simulink model "sedemo_DVS_model"  (Simulink 7.5)
settings: Solver=VariableStepDiscrete  StartTime=0.0  StopTime=inf  MaxStep=inf  RelTol=1e-3
undefined symbols (not defined in the file or in its folder): des_subsystemblock, des_subsysteminport, des_subsystemoutport, des_subsystemsupportblock, sedemo_DVS_gain_fcn, sedemo_DVS_init_fcn
libraries: simeventstranslate1 x3, simeventsgenerators1 x3, simulink x2, simeventssignalmanage1 x2, simeventstiming1 x2, simeventssink1 x1, simeventsqueue1 x1, simeventsserver1 x1, simeventsgates1 x1
settings Model: Creator=The MathWorks Inc.  ExtModeAutoUpdateStatusClock=off
settings DataIOCC: SaveOutput=off  SignalLogging=off  SaveTime=off
settings OptimizationCC: InitFltsAndDblsToZero=on
settings DebuggingCC: AlgebraicLoopMsg=error  SaveWithParameterizedLinksMsg=none  SignalResolutionControl=TryResolveAllWithWarning  SolverPrmCheckMsg=none  MultiTaskDSMMsg=warning  MultiTaskCondExecSysMsg=none  StrictBusMsg=Warning
settings RTWCC: IncludeERTFirstTime=on
settings GRTTargetCC: TargetFcnLib=ansi_tfl_tmw.mat
settings SimEventsCC: propIdentEventSeed=12345678  propDiagAttribOutput=1  propDiagFcnCallOutput=1  propDiagStatOutput=0

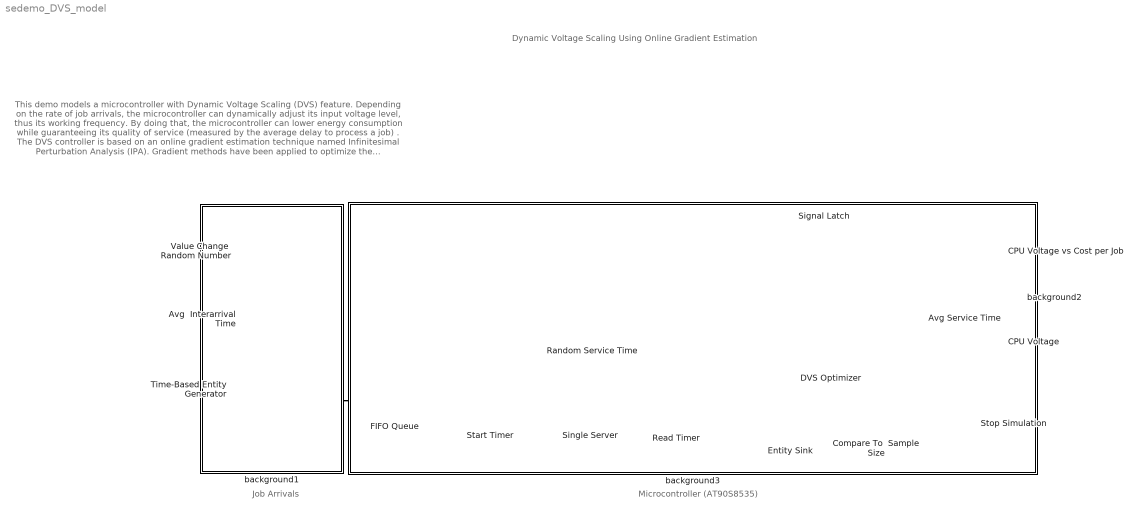
== system sedemo_DVS_model ==
  note: Job Arrivals
  note: Microcontroller (AT90S8535)
  note: Dynamic Voltage Scaling Using Online Gradient Estimation
  note: This demo models a microcontroller with Dynamic Voltage Scaling (DVS) feature. Depending on the rate of job arrivals, the microcontroller can dynamically
      | adjust its input voltage level, thus its working frequency. By doing that, the microcontroller can lower energy consumption while guaranteeing its quality
      | of service (measured by the average delay to process a job) .
      |
      | The DVS controller is based on an online gradient estimation technique named Infinitesimal Perturbation Analysis (IPA). Gradient methods have been applied
      | to optimize the performance of the microcontroller.
      |
      | During the simulation, observe how the DVS controller finds the optimal input voltage. Try changing the Avg Interarrival Time to values between 0.15 and
      | 3.0 when running the model.
  Avg  Interarrival Time : Subsystem  LoadFcn=slideg Load  InitFcn=|  StartFcn=slideg StartFcn  StopFcn=slideg StopFcn  mask(Slider Gain){low=0.15, gain=0.26, high=3}
      | global int_arr;                        
      | int_arr=str2num(get_param(gcb,'gain'));
      settings: CopyFcn=slideg Copy  DeleteFcn=slideg DeleteBlock  NameChangeFcn=slideg NameChange  OpenFcn=slideg Open  CloseFcn=slideg Close  ParentCloseFcn=slideg ParentClose
      mask Display: disp(gain)
  Avg Service Time : Display
  CPU Voltage : Display
  CPU Voltage vs Cost per Job : MATLABFcn  LoadFcn=|  StartFcn=sedemo_DVS_init_fcn;  MATLABFcn=sedemo_DVS_plot_fcn  OutputDimensions=0
      | global FigureHdl;
      | FigureHdl=1;
      settings: ModelCloseFcn=|
      | global FigureHdl;
      | figure(FigureHdl);
      | close(FigureHdl);
      | clear tout;
      | clear global FigureHdl;
      | clear int_arr;
  Compare To  Sample Size : simulink/Logic and Bit Operations/Compare To Constant  SystemSampleTime=-1  relop=>  const=5000  LogicOutDataTypeMode=boolean  ZeroCross=off
  DVS Optimizer : Subsystem
  Entity Sink : simeventssink1/Entity Sink  Priority=1  SystemSampleTime=-1  AvailableForArrivals=on  StatNumberArrived=On
  FIFO Queue : simeventsqueue1/FIFO Queue  Priority=1  SystemSampleTime=-1  Capacity=1e10  EnableTOPort=off  StatNumberDeparted=Off  StatNumberInBlock=On  StatPendingEntity=Off  StatAverageWait=Off  StatAverageQueueLength=Off  StatNumberTimedout=Off
  Random Service Time : Subsystem
  Read Timer : simeventstiming1/Read Timer  Priority=0  SystemSampleTime=-1  TimerTag=T1  TimerModeOption=Error  TimerStop=off  StatNumberDeparted=On  StatTimerNumberDeparted=Off  StatTimeElapsed=On  StatAverageTimeElapsed=Off
  Signal Latch : simeventssignalmanage1/Signal Latch  Priority=1  SystemSampleTime=-1  InitialMemoryValue=0.125  WriteMemoryUpon=Change in signal from port wvc  MemoryWriteEdgeOption=Either  SpecifyWriteEventPriority=off  PriorityMemoryWrite=7100  ReadMemoryUpon=Write to memory event  MemoryReadEdgeOption=Falling  SpecifyReadEventPriority=on  PriorityMemoryRead=7000  ReportMemoryState=off  ReportMemoryUponWrite=off  ReportMemoryUponRead=on
  Single Server : simeventsserver1/Single Server  Priority=1  SystemSampleTime=-1  ServiceTimeFrom=Signal port t  ServiceTime=1  AttributeName=ServiceTime  PriorityServiceCompletion=500  PermitPreemption=off  SortingAttributeName=PriorityAttributeName  SortingDirection=Ascending  WriteToAttribute=off  ResidualAttributeName=ResidualServiceTime  CreateAttribute=on  EnableTOPort=off  StatNumberDeparted=Off  StatNumberInBlock=Off  StatNumberPreempted=Off  StatPendingEntity=Off  StatAverageWait=Off  StatUtilization=Off  StatNumberTimedout=Off
  Start Timer : simeventstiming1/Start Timer  Priority=0  SystemSampleTime=-1  TimerTag=T1  TimerStartedOption=Warn and continue  StatNumberDeparted=On
  Stop Simulation : Stop
  Time-Based Entity Generator : simeventsgenerators1/Entity Generators/Time-Based Entity Generator  Priority=1  DialogController=des_ddg_create  DialogControllerArgs=DataTag18  SystemSampleTime=-1  GenerateEntitiesUpon=Intergeneration time from port t  Distribution=Constant  Minimum=0  Maximum=1  Mean=1  InitialSeed=12345  Period=1  PriorityEntityGeneration=300  GenerateEntityAtSimulationStart=off  ResponseWhenBlocked=Pause generation  ResponseWhenUnblocked=Immediate restart  EntityType=Standard  StatNumberDeparted=On  StatPendingEntity=Off  StatAverageIntergenerationTime=Off
  Value Change  Random Number : Subsystem
  background1 : Subsystem
      mask Display: disp('')
  background2 : Subsystem
      mask Display: disp('')
  background3 : Subsystem
      mask Display: disp('')
  wires:
  Read Timer/1 -> DVS Optimizer/3(#d)
  DVS Optimizer/2(voltage) -> CPU Voltage/1
  Signal Latch/1 -> DVS Optimizer/2(theta0), Random Service Time/1(in)
  DVS Optimizer/1(theta1) -> Avg Service Time/1, Signal Latch/2, Signal Latch/1, CPU Voltage vs Cost per Job/1
  FIFO Queue/1 -> DVS Optimizer/1(QState)
  Value Change  Random Number/1(out) -> Avg  Interarrival Time/1(In1)
  Random Service Time/1(out) -> Single Server/1
  Read Timer/2 -> DVS Optimizer/4(et)
  Start Timer/1 -> Random Service Time/2(vc)
  Entity Sink/1 -> Compare To  Sample Size/1
  Avg  Interarrival Time/1(Out1) -> Time-Based Entity Generator/1
  Time-Based Entity Generator/1 -> Value Change  Random Number/1(vc)
  Compare To  Sample Size/1 -> Stop Simulation/1
  connections:
  FIFO Queue/RConn1 -- Start Timer/LConn1
  Start Timer/RConn1 -- Single Server/LConn1
  Single Server/RConn1 -- Read Timer/LConn1
  Read Timer/RConn1 -- Entity Sink/LConn1
  Time-Based Entity Generator/RConn1 -- FIFO Queue/LConn1

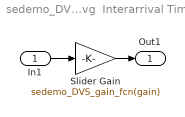
== system sedemo_DVS_model/Avg  Interarrival Time ==
  In1 : Inport  OutDataType=sfix(16)  OutScaling=2^0
  Slider Gain : Gain  Gain=sedemo_DVS_gain_fcn(gain)  ParameterDataType=sfix(16)  ParameterScaling=2^0  OutDataType=sfix(16)  OutScaling=2^0  SaturateOnIntegerOverflow=on  OutDataTypeStr=Inherit: Same as input  ParamDataTypeStr=Inherit: Same as input
  Out1 : Outport  OutDataType=sfix(16)  OutScaling=2^0
  wires:
  Slider Gain/1 -> Out1/1
  In1/1 -> Slider Gain/1

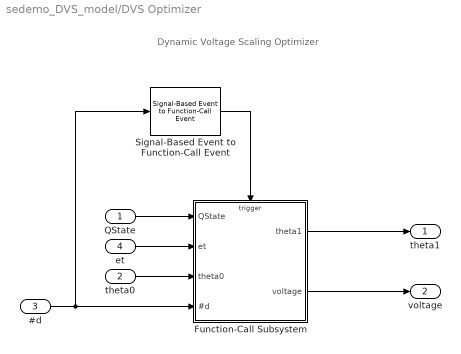
== system sedemo_DVS_model/DVS Optimizer ==
  note: Dynamic Voltage Scaling Optimizer
  QState : Inport  OutDataType=sfix(16)  OutScaling=2^0
  theta0 : Inport  Port=2  OutDataType=sfix(16)  OutScaling=2^0
  #d : Inport  Port=3  OutDataType=sfix(16)  OutScaling=2^0
  et : Inport  Port=4  OutDataType=sfix(16)  OutScaling=2^0
  Function-Call Subsystem : Subsystem  TreatAsAtomicUnit=on
      settings: PropExecContextOutsideSubsystem=on
  Signal-Based Event to Function-Call Event : simeventstranslate1/Signal-Based Event to Function-Call Event  Priority=1  SystemSampleTime=-1  GenerateFunctionCallUpon=Change in signal from port vc  SignalEdgeOption=Rising  EnableE1Port=off  EnableF2Port=off  EnableE2Port=off  SpecifyEventPriority=off  PriorityFunctionCall=200  FunctionCallDelayFrom=Dialog  DelayFunctionCall=0  StatNumberF1Calls=Off  StatNumberF2Calls=Off
  theta1 : Outport  OutDataType=sfix(16)  OutScaling=2^0
  voltage : Outport  Port=2  OutDataType=sfix(16)  OutScaling=2^0
  wires:
  Signal-Based Event to Function-Call Event/1 -> Function-Call Subsystem/Trigger
  #d/1 -> Signal-Based Event to Function-Call Event/1, Function-Call Subsystem/4(#d)
  QState/1 -> Function-Call Subsystem/1(QState)
  et/1 -> Function-Call Subsystem/2(et)
  theta0/1 -> Function-Call Subsystem/3(theta0)
  Function-Call Subsystem/1(theta1) -> theta1/1
  Function-Call Subsystem/2(voltage) -> voltage/1

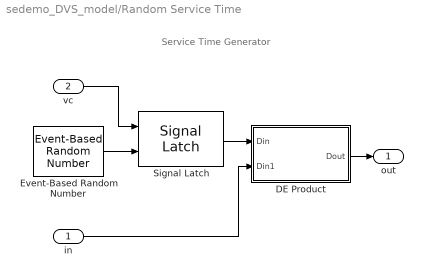
== system sedemo_DVS_model/Random Service Time ==
  note: Service Time Generator
  in : Inport  OutDataType=sfix(16)  OutScaling=2^0
  vc : Inport  Port=2  OutDataType=sfix(16)  OutScaling=2^0
  DE Product : Subsystem  LoadFcn=des_subsystemblock(gcb, 'load');  InitFcn=des_subsystemblock(gcb, 'init');  StartFcn=des_subsystemblock(gcb, 'start');  StopFcn=des_subsystemblock(gcb, 'stop');
      settings: CopyFcn=des_subsystemblock(gcb, 'copy');  DeleteFcn=des_subsystemblock(gcb, 'delete');  UndoDeleteFcn=des_subsystemblock(gcb, 'undodelete');  ModelCloseFcn=des_subsystemblock(gcb, 'modelclose');  PreSaveFcn=des_subsystemblock(gcb, 'presave');  NameChangeFcn=des_subsystemblock(gcb, 'namechange');  OpenFcn=des_subsystemblock(gcb, 'open');  ParentCloseFcn=des_subsystemblock(gcb, 'parentclose');  ErrorFcn=des_subsystemerror
      mask Type: Discrete Event Subsystem
      mask Help: helpview(simeventsbhelp);
  Event-Based Random Number : simeventsgenerators1/Signal Generators/Event-Based Random Number  SystemSampleTime=-1  distribution=Exponential  meanExp=1  minUnif=0  maxUnif=1  pOneBern=0.25  pSuccessBino=0.5  numTrialBino=1  meanNorm=0  stdNorm=1  minTri=1  maxTri=3  modeTri=2  thresholdLogn=0  scaleLogn=1  shapeLogn=1  pSuccessGeo=0.5  meanPoiss=1  thresholdLogl=0  scaleLogl=1  thresholdGam=0  scaleGam=1  shapeGam=1  minBeta=0  maxBeta=1  shape1Beta=1  shape2Beta=1  minUnid=0  maxUnid=1  numValueUnid=2  thresholdWbl=0  scaleWbl=1  shapeWbl=1  valueVecCont=[0 1]  cdfVecCont=[0 1]  valueVecDisc=[0 1]  probVecDisc=[0.5 0.5]  seed=35467  IsProcessed=on  isConnected=1
  Signal Latch : simeventssignalmanage1/Signal Latch  Priority=1  SystemSampleTime=-1  InitialMemoryValue=.22  WriteMemoryUpon=Change in signal from port wvc  MemoryWriteEdgeOption=Rising  SpecifyWriteEventPriority=on  PriorityMemoryWrite=7100  ReadMemoryUpon=Write to memory event  MemoryReadEdgeOption=Falling  SpecifyReadEventPriority=on  PriorityMemoryRead=7000  ReportMemoryState=off  ReportMemoryUponWrite=off  ReportMemoryUponRead=on
  out : Outport  OutDataType=sfix(16)  OutScaling=2^0
  wires:
  DE Product/1(Dout) -> out/1
  Event-Based Random Number/1 -> Signal Latch/2
  vc/1 -> Signal Latch/1
  Signal Latch/1 -> DE Product/1(Din)
  in/1 -> DE Product/2(Din1)

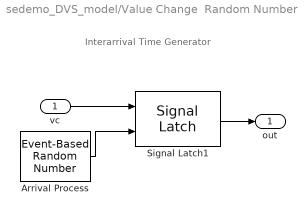
== system sedemo_DVS_model/Value Change  Random Number ==
  note: Interarrival Time Generator
  vc : Inport  OutDataType=sfix(16)  OutScaling=2^0
  Arrival Process : simeventsgenerators1/Signal Generators/Event-Based Random Number  SystemSampleTime=-1  distribution=Exponential  meanExp=1  minUnif=0  maxUnif=1  pOneBern=0.25  pSuccessBino=0.5  numTrialBino=1  meanNorm=0  stdNorm=1  minTri=1  maxTri=3  modeTri=2  thresholdLogn=0  scaleLogn=1  shapeLogn=1  pSuccessGeo=0.5  meanPoiss=1  thresholdLogl=0  scaleLogl=1  thresholdGam=0  scaleGam=1  shapeGam=1  minBeta=0  maxBeta=1  shape1Beta=1  shape2Beta=1  minUnid=0  maxUnid=1  numValueUnid=2  thresholdWbl=0  scaleWbl=1  shapeWbl=1  valueVecCont=[0 1]  cdfVecCont=[0 1]  valueVecDisc=[0 1]  probVecDisc=[0.5 0.5]  seed=98765  IsProcessed=on  isConnected=1
  Signal Latch1 : simeventsgates1/Signal Latch  Priority=1  SystemSampleTime=-1  InitialMemoryValue=0.45  WriteMemoryUpon=Change in signal from port wvc  MemoryWriteEdgeOption=Rising  SpecifyWriteEventPriority=on  PriorityMemoryWrite=7100  ReadMemoryUpon=Write to memory event  MemoryReadEdgeOption=Falling  SpecifyReadEventPriority=on  PriorityMemoryRead=7000  ReportMemoryState=off  ReportMemoryUponWrite=off  ReportMemoryUponRead=on
  out : Outport  OutDataType=sfix(16)  OutScaling=2^0
  wires:
  Arrival Process/1 -> Signal Latch1/2
  vc/1 -> Signal Latch1/1
  Signal Latch1/1 -> out/1

== system sedemo_DVS_model/background1 ==

== system sedemo_DVS_model/background2 ==

== system sedemo_DVS_model/background3 ==

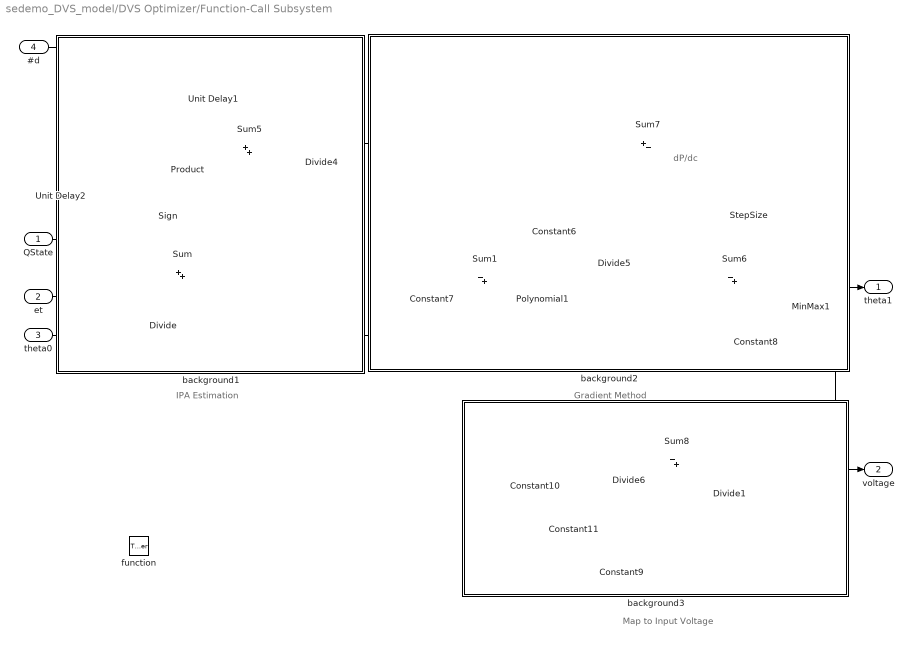
== system sedemo_DVS_model/DVS Optimizer/Function-Call Subsystem ==
  note: Map to Input Voltage
  note: dP/dc
  note: Gradient Method
  note: IPA Estimation
  QState : Inport  OutDataType=sfix(16)  OutScaling=2^0
  et : Inport  Port=2  OutDataType=sfix(16)  OutScaling=2^0
  theta0 : Inport  Port=3  OutDataType=sfix(16)  OutScaling=2^0
  #d : Inport  Port=4  OutDataType=sfix(16)  OutScaling=2^0
  function : TriggerPort  TriggerType=function-call
  Constant10 : Constant  Value=1/12  OutDataType=sfix(16)  OutScaling=2^0
  Constant11 : Constant  OutDataType=sfix(16)  OutScaling=2^0
  Constant6 : Constant  Value=1/36  OutDataType=sfix(16)  OutScaling=2^0
  Constant7 : Constant  Value=1/12  OutDataType=sfix(16)  OutScaling=2^0
  Constant8 : Constant  Value=0.12  OutDataType=sfix(16)  OutScaling=2^0
  Constant9 : Constant  Value=2  OutDataType=sfix(16)  OutScaling=2^0
  Divide : Product  Inputs=*/  OutDataType=sfix(16)  OutScaling=2^-10
  Divide1 : Product  Inputs=/*  OutDataType=sfix(16)  OutScaling=2^-10
  Divide4 : Product  Inputs=/*  OutDataType=sfix(16)  OutScaling=2^-10
  Divide5 : Product  Inputs=**/  OutDataType=sfix(16)  OutScaling=2^-10
  Divide6 : Product  Inputs=/*  OutDataType=sfix(16)  OutScaling=2^-10
  MinMax1 : MinMax  Function=max  Inputs=2  OutDataType=sfix(16)  OutScaling=2^0
  Polynomial1 : simulink/Math Operations/Polynomial  coefs=[1,0,0,0]
  Product : Product  OutDataType=sfix(16)  OutScaling=2^0  RndMeth=Zero
  Sign : Signum
  StepSize : Gain  Gain=1e-5  ParameterDataType=sfix(16)  ParameterScaling=2^0  OutDataType=sfix(16)  OutScaling=2^0
  Sum : Sum  Inputs=|++  OutDataType=sfix(16)  OutScaling=2^0
  Sum1 : Sum  Inputs=|-+  OutDataType=sfix(16)  OutScaling=2^0
  Sum5 : Sum  Inputs=|++  OutDataType=sfix(16)  OutScaling=2^0
  Sum6 : Sum  Inputs=|-+  OutDataType=sfix(16)  OutScaling=2^0
  Sum7 : Sum  Inputs=|+-  OutDataType=sfix(16)  OutScaling=2^0
  Sum8 : Sum  Inputs=|-+  OutDataType=sfix(16)  OutScaling=2^0
  Unit Delay1 : UnitDelay  SampleTime=-1
  Unit Delay2 : UnitDelay  SampleTime=-1
  background1 : Subsystem
      mask Display: disp('')
  background2 : Subsystem
      mask Display: disp('')
  background3 : Subsystem
      mask Display: disp('')
  theta1 : Outport  OutDataType=sfix(16)  OutScaling=2^0  InitialOutput=0.125
  voltage : Outport  Port=2  OutDataType=sfix(16)  OutScaling=2^0  InitialOutput=6
  wires:
  Divide1/1 -> voltage/1
  Constant9/1 -> Divide1/2
  Sum8/1 -> Divide1/1
  Constant11/1 -> Sum8/2
  Divide6/1 -> Sum8/1
  Constant10/1 -> Divide6/2
  MinMax1/1 -> theta1/1, Divide6/1
  Divide5/1 -> Sum7/2
  Sum7/1 -> StepSize/1
  Constant7/1 -> Sum1/1
  Sum1/1 -> Polynomial1/1
  Polynomial1/1 -> Divide5/3
  Constant6/1 -> Divide5/1
  Divide4/1 -> Sum7/1
  Sum5/1 -> Unit Delay1/1, Divide4/2
  Unit Delay1/1 -> Sum5/1
  theta0/1 -> Divide5/2, Sum1/2, Sum6/2, Divide/2
  Sum/1 -> Sum5/2, Product/1
  Unit Delay2/1 -> Sum/1
  Product/1 -> Unit Delay2/1
  QState/1 -> Sign/1
  Sign/1 -> Product/2
  et/1 -> Divide/1
  Divide/1 -> Sum/2
  #d/1 -> Divide4/1
  StepSize/1 -> Sum6/1
  Constant8/1 -> MinMax1/2
  Sum6/1 -> MinMax1/1

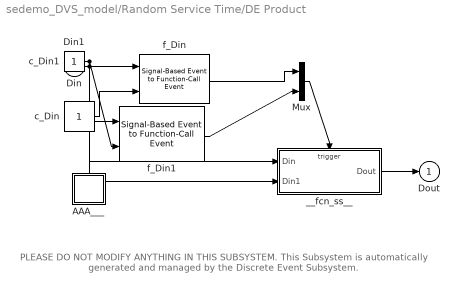
== system sedemo_DVS_model/Random Service Time/DE Product ==
  note: PLEASE DO NOT MODIFY ANYTHING IN THIS SUBSYSTEM.
      | This Subsystem is automatically generated and
      | managed by the Discrete Event Subsystem.
  Din : Inport  PortDimensions=1  DataType=double  OutDataType=sfix(16)  OutScaling=2^0  OutDataTypeStr=double
  Din1 : Inport  Port=2  PortDimensions=1  DataType=double  OutDataType=sfix(16)  OutScaling=2^0  OutDataTypeStr=double
  AAA___ : Subsystem  LoadFcn=des_subsystemsupportblock(gcb, 'load');  InitFcn=des_subsystemsupportblock(gcb, 'init');  StartFcn=des_subsystemsupportblock(gcb, 'start');  StopFcn=des_subsystemsupportblock(gcb, 'stop');
      settings: CopyFcn=des_subsystemsupportblock(gcb, 'copy');  DeleteFcn=des_subsystemsupportblock(gcb, 'delete');  UndoDeleteFcn=des_subsystemsupportblock(gcb, 'undodelete');  ModelCloseFcn=des_subsystemsupportblock(gcb, 'modelclose');  PreSaveFcn=des_subsystemsupportblock(gcb, 'presave');  NameChangeFcn=des_subsystemsupportblock(gcb, 'namechange');  OpenFcn=des_subsystemsupportblock(gcb, 'open');  ParentCloseFcn=des_subsystemsupportblock(gcb, 'parentclose');
  Mux : Mux  Inputs=2
  __fcn_ss__ : Subsystem  TreatAsAtomicUnit=on
      settings: PropExecContextOutsideSubsystem=on
  c_Din : Constant  OutDataType=sfix(16)  OutScaling=2^0
  c_Din1 : Constant  OutDataType=sfix(16)  OutScaling=2^0
  f_Din : simeventstranslate1/Signal-Based Event to Function-Call Event  Priority=1  SystemSampleTime=-1  GenerateFunctionCallUpon=Sample time hit from port ts  SignalEdgeOption=Rising  EnableE1Port=on  EnableF2Port=off  EnableE2Port=off  SpecifyEventPriority=off  PriorityFunctionCall=20  FunctionCallDelayFrom=Dialog  DelayFunctionCall=0  StatNumberF1Calls=Off  StatNumberF2Calls=Off  MaskBlockType=none
  f_Din1 : simeventstranslate1/Signal-Based Event to Function-Call Event  Priority=1  SystemSampleTime=-1  GenerateFunctionCallUpon=Sample time hit from port ts  SignalEdgeOption=Rising  EnableE1Port=on  EnableF2Port=off  EnableE2Port=off  SpecifyEventPriority=off  PriorityFunctionCall=20  FunctionCallDelayFrom=Dialog  DelayFunctionCall=0  StatNumberF1Calls=Off  StatNumberF2Calls=Off  MaskBlockType=none
  Dout : Outport  OutDataType=sfix(16)  OutScaling=2^0
  wires:
  __fcn_ss__/1(Dout) -> Dout/1
  f_Din/1 -> Mux/1
  c_Din/1 -> f_Din/2
  Mux/1 -> __fcn_ss__/Trigger
  f_Din1/1 -> Mux/2
  c_Din1/1 -> f_Din1/2
  Din/1 -> f_Din/1, __fcn_ss__/1(Din)
  Din1/1 -> f_Din1/1, __fcn_ss__/2(Din1)

== system sedemo_DVS_model/DVS Optimizer/Function-Call Subsystem/background1 ==

== system sedemo_DVS_model/DVS Optimizer/Function-Call Subsystem/background2 ==

== system sedemo_DVS_model/DVS Optimizer/Function-Call Subsystem/background3 ==

== system sedemo_DVS_model/Random Service Time/DE Product/AAA___ ==

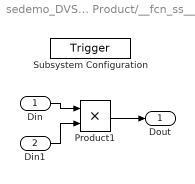
== system sedemo_DVS_model/Random Service Time/DE Product/__fcn_ss__ ==
  Din : Inport  LoadFcn=des_subsysteminport(gcb, 'load');  InitFcn=des_subsysteminport(gcb, 'init');  StartFcn=des_subsysteminport(gcb, 'start');  StopFcn=des_subsysteminport(gcb, 'stop');  OutDataType=sfix(16)  OutScaling=2^0  mask(Discrete Event Inport){PermitSubsystemEvents=on, TypeOfEvent=Sample time hit, SignalEdgeOption=Rising, SpecifyEventPriority=off, PrioritySubsystemEvent=20}
      mask prompts: PermitSubsystemEvents "Execute subsystem upon signal-based events"; TypeOfEvent "Type of signal-based event:"; SignalEdgeOption "Type of change in signal value:"; SpecifyEventPriority "Specify event priority for executing subsystem"; PrioritySubsystemEvent "Subsystem execution event priority:"
      mask help: Input port for a Discrete Event Subsystem block. This block can conditionally execute the subsystem upon signal-based events that meet specified criteria.
      mask init:
      | des_subsystemmask(gcb, 'init','apply')
      settings: CopyFcn=des_subsysteminport(gcb, 'copy');  DeleteFcn=des_subsysteminport(gcb, 'delete');  UndoDeleteFcn=des_subsysteminport(gcb, 'undodelete');  ModelCloseFcn=des_subsysteminport(gcb, 'modelclose');  PreSaveFcn=des_subsysteminport(gcb, 'presave');  NameChangeFcn=des_subsysteminport(gcb, 'namechange');  ParentCloseFcn=des_subsysteminport(gcb, 'parentclose');
      mask Help: helpview(simeventsbhelp);
      mask StyleString: checkbox,popup(Change in signal|Trigger|Sample time hit),popup(Rising|Falling|Either),checkbox,edit
      mask CallbackString: des_subsystemmask(gcb, 'cbPermitSubsystemEvents', 'noapply');|des_subsystemmask(gcb,'cbTypeOfEvent','noapply');||des_subsystemmask(gcb, 'cbSpecifyEventPriority', 'noapply');|
  Din1 : Inport  LoadFcn=des_subsysteminport(gcb, 'load');  InitFcn=des_subsysteminport(gcb, 'init');  StartFcn=des_subsysteminport(gcb, 'start');  StopFcn=des_subsysteminport(gcb, 'stop');  Port=2  OutDataType=sfix(16)  OutScaling=2^0  mask(Discrete Event Inport){PermitSubsystemEvents=on, TypeOfEvent=Sample time hit, SignalEdgeOption=Rising, SpecifyEventPriority=off, PrioritySubsystemEvent=20}
      mask prompts: PermitSubsystemEvents "Execute subsystem upon signal-based events"; TypeOfEvent "Type of signal-based event:"; SignalEdgeOption "Type of change in signal value:"; SpecifyEventPriority "Specify event priority for executing subsystem"; PrioritySubsystemEvent "Subsystem execution event priority:"
      mask help: Input port for a Discrete Event Subsystem block. This block can conditionally execute the subsystem upon signal-based events that meet specified criteria.
      mask init:
      | des_subsystemmask(gcb, 'init','apply')
      settings: CopyFcn=des_subsysteminport(gcb, 'copy');  DeleteFcn=des_subsysteminport(gcb, 'delete');  UndoDeleteFcn=des_subsysteminport(gcb, 'undodelete');  ModelCloseFcn=des_subsysteminport(gcb, 'modelclose');  PreSaveFcn=des_subsysteminport(gcb, 'presave');  NameChangeFcn=des_subsysteminport(gcb, 'namechange');  ParentCloseFcn=des_subsysteminport(gcb, 'parentclose');
      mask Help: helpview(simeventsbhelp);
      mask StyleString: checkbox,popup(Change in signal|Trigger|Sample time hit),popup(Rising|Falling|Either),checkbox,edit
      mask CallbackString: des_subsystemmask(gcb, 'cbPermitSubsystemEvents', 'noapply');|des_subsystemmask(gcb,'cbTypeOfEvent','noapply');||des_subsystemmask(gcb, 'cbSpecifyEventPriority', 'noapply');|
  Subsystem Configuration : TriggerPort  TriggerType=function-call
      settings: CopyFcn=des_subsystemconfigblock(gcb, 'copy');  DeleteFcn=des_subsystemconfigblock(gcb, 'delete');  UndoDeleteFcn=des_subsystemconfigblock(gcb, 'undodelete');
      mask Type: Subsystem Configuration
      mask Description: Configuration for a Discrete Event Subsystem block. Every discrete event subsystem window must contain exactly one copy of this configuration block. Do not delete this block.
      mask Help: helpview(simeventsbhelp);
      mask Display: disp('Do Not Delete');
  Product1 : Product  OutDataType=sfix(16)  OutScaling=2^0  RndMeth=Zero
  Dout : Outport  LoadFcn=des_subsystemoutport(gcb, 'load');  InitFcn=des_subsystemoutport(gcb, 'init');  StartFcn=des_subsystemoutport(gcb, 'start');  StopFcn=des_subsystemoutport(gcb, 'stop');  OutDataType=sfix(16)  OutScaling=2^0
      settings: CopyFcn=des_subsystemoutport(gcb, 'copy');  DeleteFcn=des_subsystemoutport(gcb, 'delete');  UndoDeleteFcn=des_subsystemoutport(gcb, 'undodelete');  ModelCloseFcn=des_subsystemoutport(gcb, 'modelclose');  PreSaveFcn=des_subsystemoutport(gcb, 'presave');  NameChangeFcn=des_subsystemoutport(gcb, 'namechange');  ParentCloseFcn=des_subsystemoutport(gcb, 'parentclose');
      mask Type: Discrete Event Outport
      mask Description: Provide an output port for a Discrete Event Subsystem block.
      mask Help: helpview(simeventsbhelp);
  wires:
  Din/1 -> Product1/1
  Din1/1 -> Product1/2
  Product1/1 -> Dout/1
